simulink model "Ex3"  (Simulink 7.8)
settings: Solver=ode45  StartTime=0.0  StopTime=10.0  RelTol=1e-3
settings Model: Creator=alex  LastModifiedBy=alex

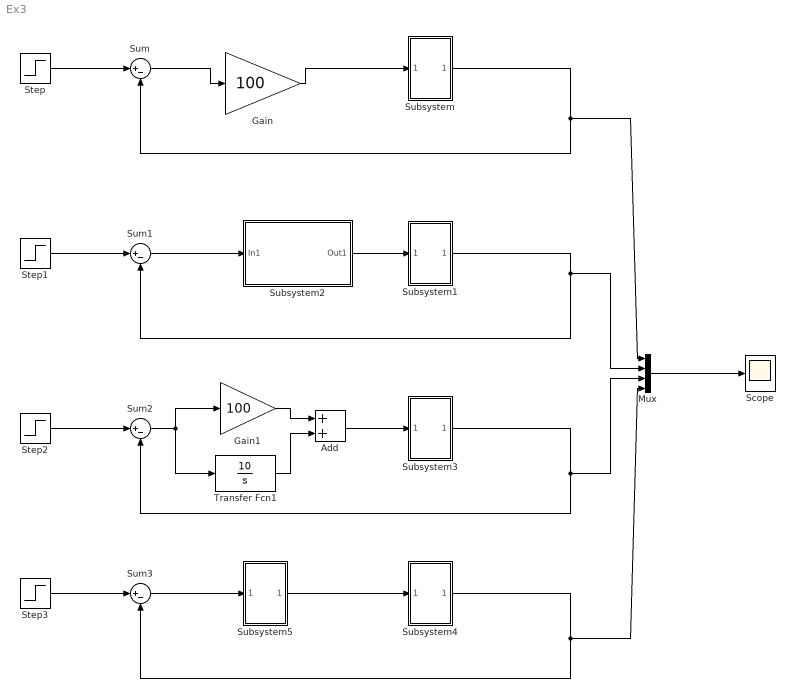
== system Ex3 ==
  Add : Sum
  Gain : Gain  Gain=100
  Gain1 : Gain  Gain=100
  Mux : Mux
  Scope : Scope
      settings: MaxDataPoints=500000  SampleInput=on
  Step{,1..3} (4 alike) : Step  SampleTime=0
  Subsystem : Subsystem
  Subsystem1 : Subsystem
  Subsystem2 : Subsystem
  Subsystem3 : Subsystem
  Subsystem4 : Subsystem
  Subsystem5 : Subsystem
  Sum{,1..3} (4 alike) : Sum  Inputs=|+-
  Transfer Fcn1 : TransferFcn  Numerator=[10]  Denominator=[1 0]
  wires:
  Subsystem/1(Out1) -> Sum/2, Mux/1
  Step/1 -> Sum/1
  Sum/1 -> Gain/1
  Gain/1 -> Subsystem/1(In1)
  Step1/1 -> Sum1/1
  Subsystem2/1(Out1) -> Subsystem1/1(In1)
  Sum1/1 -> Subsystem2/1(In1)
  Subsystem3/1(Out1) -> Sum2/2, Mux/3
  Step2/1 -> Sum2/1
  Add/1 -> Subsystem3/1(In1)
  Transfer Fcn1/1 -> Add/2
  Gain1/1 -> Add/1
  Sum2/1 -> Transfer Fcn1/1, Gain1/1
  Subsystem4/1(Out1) -> Sum3/2, Mux/4
  Step3/1 -> Sum3/1
  Subsystem5/1(Out1) -> Subsystem4/1(In1)
  Sum3/1 -> Subsystem5/1(In1)
  Subsystem1/1(Out1) -> Sum1/2, Mux/2
  Mux/1 -> Scope/1

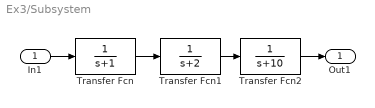
== system Ex3/Subsystem ==
  In1 : Inport
  Transfer Fcn : TransferFcn  Denominator=[1 1]
  Transfer Fcn1 : TransferFcn  Denominator=[1 2]
  Transfer Fcn2 : TransferFcn  Denominator=[1 10]
  Out1 : Outport
  wires:
  Transfer Fcn1/1 -> Transfer Fcn2/1
  Transfer Fcn/1 -> Transfer Fcn1/1
  In1/1 -> Transfer Fcn/1
  Transfer Fcn2/1 -> Out1/1

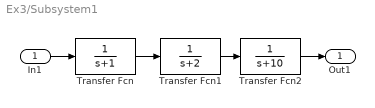
== system Ex3/Subsystem1 ==
  In1 : Inport
  Transfer Fcn : TransferFcn  Denominator=[1 1]
  Transfer Fcn1 : TransferFcn  Denominator=[1 2]
  Transfer Fcn2 : TransferFcn  Denominator=[1 10]
  Out1 : Outport
  wires:
  Transfer Fcn1/1 -> Transfer Fcn2/1
  Transfer Fcn/1 -> Transfer Fcn1/1
  In1/1 -> Transfer Fcn/1
  Transfer Fcn2/1 -> Out1/1

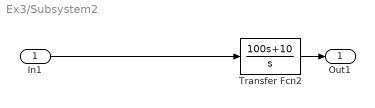
== system Ex3/Subsystem2 ==
  In1 : Inport
  Transfer Fcn2 : TransferFcn  Numerator=[100 10]  Denominator=[1 0]
  Out1 : Outport
  wires:
  In1/1 -> Transfer Fcn2/1
  Transfer Fcn2/1 -> Out1/1

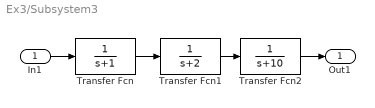
== system Ex3/Subsystem3 ==
  In1 : Inport
  Transfer Fcn : TransferFcn  Denominator=[1 1]
  Transfer Fcn1 : TransferFcn  Denominator=[1 2]
  Transfer Fcn2 : TransferFcn  Denominator=[1 10]
  Out1 : Outport
  wires:
  Transfer Fcn1/1 -> Transfer Fcn2/1
  Transfer Fcn/1 -> Transfer Fcn1/1
  In1/1 -> Transfer Fcn/1
  Transfer Fcn2/1 -> Out1/1

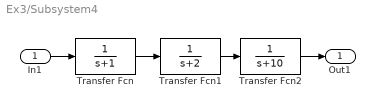
== system Ex3/Subsystem4 ==
  In1 : Inport
  Transfer Fcn : TransferFcn  Denominator=[1 1]
  Transfer Fcn1 : TransferFcn  Denominator=[1 2]
  Transfer Fcn2 : TransferFcn  Denominator=[1 10]
  Out1 : Outport
  wires:
  Transfer Fcn1/1 -> Transfer Fcn2/1
  Transfer Fcn/1 -> Transfer Fcn1/1
  In1/1 -> Transfer Fcn/1
  Transfer Fcn2/1 -> Out1/1

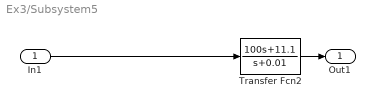
== system Ex3/Subsystem5 ==
  In1 : Inport
  Transfer Fcn2 : TransferFcn  Numerator=[100 11.1]  Denominator=[1 0.01]
  Out1 : Outport
  wires:
  In1/1 -> Transfer Fcn2/1
  Transfer Fcn2/1 -> Out1/1
